simulink model "SingleTrack3States"  (R2018a)
settings: Solver=ode4  StartTime=0.0  StopTime=10.0  FixedStep=.001  RelTol=1e-3
values from neighbouring files (symbols this model uses):
  car = Porsche911    [init.m]
  initBeta = 0    [init.m]
  initR = 0    [init.m]
  initV = 10    [init.m]
settings Model: Creator=efrem  LastModifiedBy=efrem

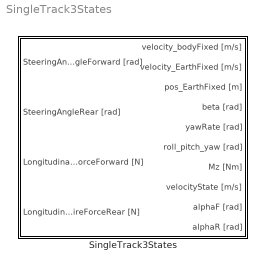
== system SingleTrack3States ==
  SingleTrack3States : Subsystem

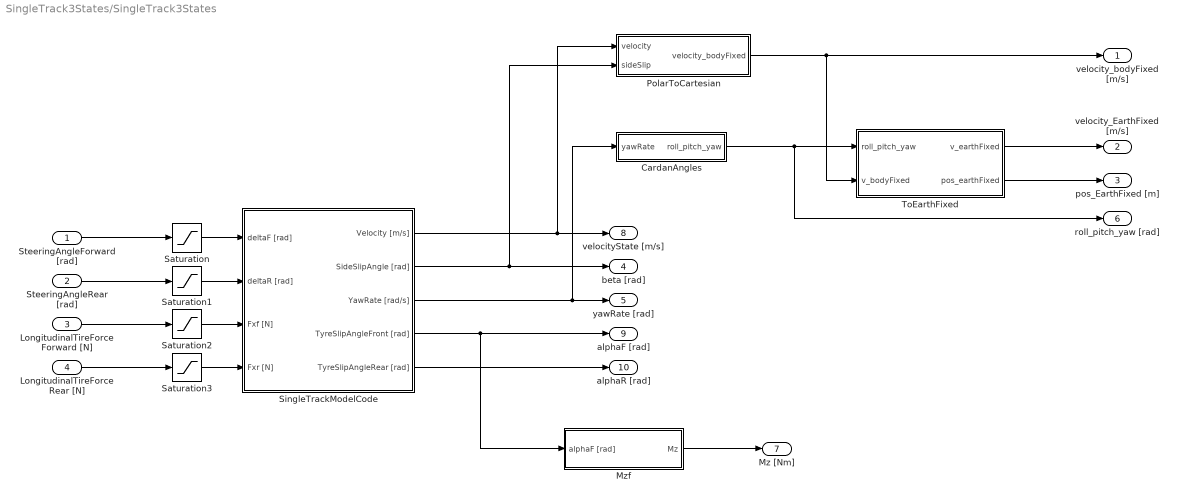
== system SingleTrack3States/SingleTrack3States ==
  SteeringAngleForward [rad] : Inport
  SteeringAngleRear [rad] : Inport  Port=2
  LongitudinalTireForceForward [N] : Inport  Port=3
  LongitudinalTireForceRear [N] : Inport  Port=4
  CardanAngles : Subsystem
  Mzf : Subsystem
  PolarToCartesian : Subsystem
  Saturation : Saturate  UpperLimit=pi/3  LowerLimit=-pi/3  ZeroCross=off
  Saturation1 : Saturate  UpperLimit=pi/3  LowerLimit=-pi/3  ZeroCross=off
  Saturation2 : Saturate  UpperLimit=10000  LowerLimit=-10000  ZeroCross=off
  Saturation3 : Saturate  UpperLimit=10000  LowerLimit=-10000  ZeroCross=off
  SingleTrackModelCode : Subsystem
  ToEarthFixed : Subsystem
  velocity_bodyFixed [m/s] : Outport
  velocity_EarthFixed [m/s] : Outport  Port=2
  pos_EarthFixed [m] : Outport  Port=3
  beta [rad] : Outport  Port=4
  yawRate [rad] : Outport  Port=5
  roll_pitch_yaw [rad] : Outport  Port=6
  Mz [Nm] : Outport  Port=7
  velocityState [m/s] : Outport  Port=8
  alphaF [rad] : Outport  Port=9
  alphaR [rad] : Outport  Port=10
  wires:
  SingleTrackModelCode/3(YawRate [rad/s]) -> CardanAngles/1(yawRate), yawRate [rad]/1
  ToEarthFixed/2(pos_earthFixed) -> pos_EarthFixed [m]/1
  PolarToCartesian/1(velocity_bodyFixed) -> ToEarthFixed/2(v_bodyFixed), velocity_bodyFixed [m/s]/1
  SingleTrackModelCode/2(SideSlipAngle [rad]) -> PolarToCartesian/2(sideSlip), beta [rad]/1
  ToEarthFixed/1(v_earthFixed) -> velocity_EarthFixed [m/s]/1
  CardanAngles/1(roll_pitch_yaw) -> roll_pitch_yaw [rad]/1, ToEarthFixed/1(roll_pitch_yaw)
  SteeringAngleForward [rad]/1 -> Saturation/1
  LongitudinalTireForceForward [N]/1 -> Saturation2/1
  LongitudinalTireForceRear [N]/1 -> Saturation3/1
  Saturation1/1 -> SingleTrackModelCode/2(deltaR [rad])
  Saturation2/1 -> SingleTrackModelCode/3(Fxf [N])
  Saturation3/1 -> SingleTrackModelCode/4(Fxr [N])
  SteeringAngleRear [rad]/1 -> Saturation1/1
  Saturation/1 -> SingleTrackModelCode/1(deltaF [rad])
  SingleTrackModelCode/1(Velocity [m/s]) -> PolarToCartesian/1(velocity), velocityState [m/s]/1
  SingleTrackModelCode/4(TyreSlipAngleFront [rad]) -> Mzf/1(alphaF [rad]), alphaF [rad]/1
  SingleTrackModelCode/5(TyreSlipAngleRear [rad]) -> alphaR [rad]/1
  Mzf/1(Mz) -> Mz [Nm]/1

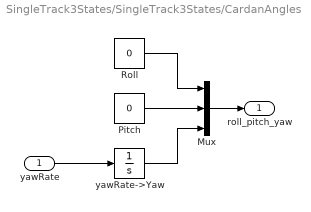
== system SingleTrack3States/SingleTrack3States/CardanAngles ==
  yawRate : Inport
  Mux : Mux  Inputs=3
  Pitch : Constant  Value=0
  Roll : Constant  Value=0
  yawRate->Yaw : Integrator
  roll_pitch_yaw : Outport
  wires:
  Roll/1 -> Mux/1
  Mux/1 -> roll_pitch_yaw/1
  Pitch/1 -> Mux/2
  yawRate->Yaw/1 -> Mux/3
  yawRate/1 -> yawRate->Yaw/1

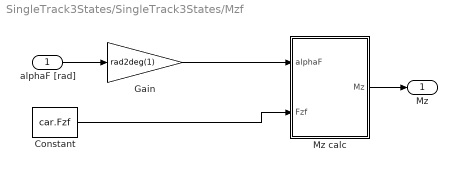
== system SingleTrack3States/SingleTrack3States/Mzf ==
  alphaF [rad] : Inport
  Constant : Constant  Value=car.Fzf
  Gain : Gain  Gain=rad2deg(1)
  Mz calc : MATLAB Function  TreatAsAtomicUnit=on
  Mz : Outport
  wires:
  Mz calc/1(Mz) -> Mz/1
  Constant/1 -> Mz calc/2(Fzf)
  Gain/1 -> Mz calc/1(alphaF)
  alphaF [rad]/1 -> Gain/1

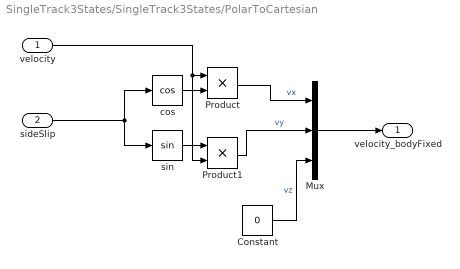
== system SingleTrack3States/SingleTrack3States/PolarToCartesian ==
  velocity : Inport
  sideSlip : Inport  Port=2
  Constant : Constant  Value=0
  Mux : Mux  Inputs=3
  Product : Product
  Product1 : Product
  cos : Trigonometry  Operator=cos
  sin : Trigonometry
  velocity_bodyFixed : Outport
  wires:
  cos/1 -> Product/2
  sin/1 -> Product1/1
  Product/1 -> Mux/1  "vx"
  velocity/1 -> Product/1, Product1/2
  Product1/1 -> Mux/2  "vy"
  sideSlip/1 -> cos/1, sin/1
  Mux/1 -> velocity_bodyFixed/1
  Constant/1 -> Mux/3  "vz"

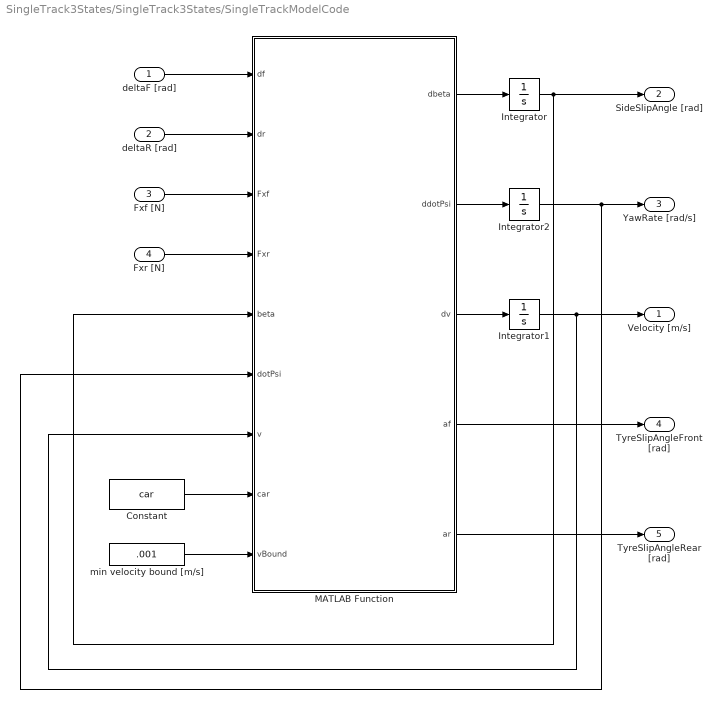
== system SingleTrack3States/SingleTrack3States/SingleTrackModelCode ==
  deltaF [rad] : Inport
  deltaR [rad] : Inport  Port=2
  Fxf [N] : Inport  Port=3
  Fxr [N] : Inport  Port=4
  Constant : Constant  Value=car  OutDataTypeStr=Bus: car_bus
  Integrator : Integrator  InitialCondition=initBeta  UpperSaturationLimit=pi/2  LowerSaturationLimit=-pi/2  ZeroCross=off
  Integrator1 : Integrator  InitialCondition=initV  UpperSaturationLimit=100  LowerSaturationLimit=0.01  IgnoreLimit=on  ZeroCross=off
  Integrator2 : Integrator  InitialCondition=initR
  MATLAB Function : MATLAB Function  TreatAsAtomicUnit=on
  min velocity bound [m/s] : Constant  Value=.001
  Velocity [m/s] : Outport
  SideSlipAngle [rad] : Outport  Port=2
  YawRate [rad/s] : Outport  Port=3
  TyreSlipAngleFront [rad] : Outport  Port=4
  TyreSlipAngleRear [rad] : Outport  Port=5
  wires:
  MATLAB Function/1(dbeta) -> Integrator/1
  MATLAB Function/2(ddotPsi) -> Integrator2/1
  MATLAB Function/3(dv) -> Integrator1/1
  Integrator/1 -> SideSlipAngle [rad]/1, MATLAB Function/5(beta)
  Integrator2/1 -> YawRate [rad/s]/1, MATLAB Function/6(dotPsi)
  Integrator1/1 -> Velocity [m/s]/1, MATLAB Function/7(v)
  deltaF [rad]/1 -> MATLAB Function/1(df)
  deltaR [rad]/1 -> MATLAB Function/2(dr)
  Fxf [N]/1 -> MATLAB Function/3(Fxf)
  Fxr [N]/1 -> MATLAB Function/4(Fxr)
  min velocity bound [m/s]/1 -> MATLAB Function/9(vBound)
  MATLAB Function/4(af) -> TyreSlipAngleFront [rad]/1
  MATLAB Function/5(ar) -> TyreSlipAngleRear [rad]/1
  Constant/1 -> MATLAB Function/8(car)

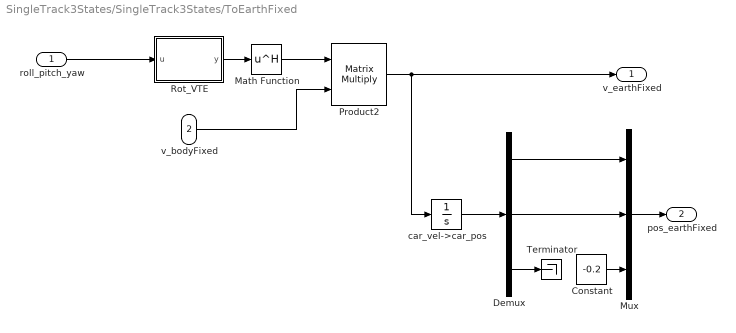
== system SingleTrack3States/SingleTrack3States/ToEarthFixed ==
  roll_pitch_yaw : Inport
  v_bodyFixed : Inport  Port=2
  Constant : Constant  Value=-0.2
  Demux : Demux  Outputs=3
  Math Function : Math  Operator=hermitian  SaturateOnIntegerOverflow=on
  Mux : Mux  Inputs=3
  Product2 : Product  Multiplication=Matrix(*)
  Rot_VTE : MATLAB Function  TreatAsAtomicUnit=on
  Terminator : Terminator
  car_vel->car_pos : Integrator
  v_earthFixed : Outport
  pos_earthFixed : Outport  Port=2
  wires:
  Rot_VTE/1(y) -> Math Function/1
  roll_pitch_yaw/1 -> Rot_VTE/1(u)
  Constant/1 -> Mux/3
  car_vel->car_pos/1 -> Demux/1
  Product2/1 -> v_earthFixed/1, car_vel->car_pos/1
  Demux/1 -> Mux/1
  Demux/2 -> Mux/2
  v_bodyFixed/1 -> Product2/2
  Mux/1 -> pos_earthFixed/1
  Math Function/1 -> Product2/1
  Demux/3 -> Terminator/1

== matlab function SingleTrack3States/ToEarthFixed/Rot_VTE ==
  data: u input; y output
function y = fcn(u)
y = Rot_VTE(u);

== matlab function SingleTrack3States/Mzf/Mz calc ==
  data: alphaF input; Mz output; Fzf input
function Mz = fcn(alphaF, Fzf)
Bz = .15;
Cz = 2.3;
Dz = -.05 * Fzf;
Ez = -10;
Mz = Dz*sin((Cz*atan(Bz*alphaF - Ez*(Bz*alphaF - atan(Bz*alphaF)))));

== matlab function SingleTrack3States/SingleTrackModelCode/MATLAB Function ==
  data: df input; dbeta output; dr input; Fxf input; Fxr input; beta input; dotPsi input; v input; car input; vBound input; ddotPsi output; dv output; af output; ar output
function [dbeta, ddotPsi, dv, af, ar] = SingleTrackModelFunctionCode(df, dr, Fxf, Fxr, beta, dotPsi, v, car, vBound)
    
    %% parse parameters 
    lf = car.LF;
    lr = car.LR;
    m = car.Mass;
    Fzf = car.Fzf;
    Fzr = car.Fzb;
    Iz = car.Iz;
    D = car.Pacejka.D;
    B = car.Pacejka.B;
    C = car.Pacejka.C;
    E = car.Pacejka.E;

    %% deadzone for the velocity
    if(v < vBound && v >= 0) 
		v = v+vBound;
	elseif (v > -vBound && v <0)
        v = v-vBound;
    end
    
    %% kinematics
    af = -atan2((v*sin(beta)+lf*dotPsi)*cos(df)-v*cos(beta)*sin(df),...
        abs((v*sin(beta)+lf*dotPsi)*sin(df)+ v*cos(beta)*cos(df)));
    
    ar = -atan2((v*sin(beta)-lr*dotPsi)*cos(dr)-v*cos(beta)*sin(dr),...
        abs((v*sin(beta)-lr*dotPsi)*sin(dr)+ v*cos(beta)*cos(dr)));
    
    af_deg = rad2deg(af);
    ar_deg = rad2deg(ar);
    
    %% Pacejka 
    Fyf = D * Fzf * sin(C * atan(B*af_deg - E*(B*af_deg - atan(B*af_deg))));
    Fyr = D * Fzr * sin(C * atan(B*ar_deg - E*(B*ar_deg - atan(B*ar_deg))));

    %% steering angle projection and vehicle dynamics
    SAP = [cos(df), -sin(df), cos(dr), -sin(dr);...
        sin(df), cos(df), sin(dr), cos(dr);...
        lf*sin(df), lf*cos(df), -lr*sin(dr), -lr*cos(dr)];

    F = [Fxf; Fyf; Fxr; Fyr];

    RotDyn = [-sin(beta), cos(beta), 0;...
        cos(beta), sin(beta), 0;...
        0, 0, 1];

    Dyn = RotDyn * (SAP * F);
    
    % parse to motions
    lat = Dyn(1);
    long = Dyn(2);
    rot = Dyn(3);
	
    dbeta = - dotPsi + lat/m/v;
    dv = long/m;
    ddotPsi = rot/Iz;

end
